simulink model "Model_1"  (R2020b)
settings: Solver=VariableStepAuto  StartTime=0.0  StopTime=200  RelTol=1e-3
settings Model: Creator=samar  LastModifiedBy=samar

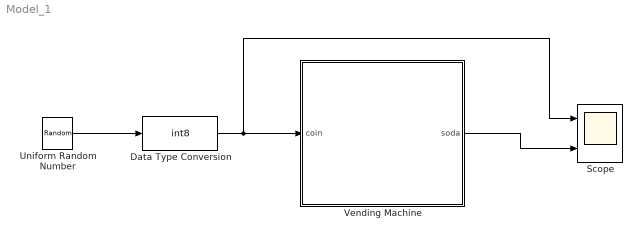
== system Model_1 ==
  Data Type Conversion : DataTypeConversion  OutDataTypeStr=int8  RndMeth=Nearest
  Scope : Scope  NumInputPorts=2
  Uniform Random Number : UniformRandomNumber  Minimum=0  Maximum=2  Seed=337  SampleTime=10
  Vending Machine : Stateflow chart  TreatAsAtomicUnit=on
  wires:
  Uniform Random Number/1 -> Data Type Conversion/1
  Data Type Conversion/1 -> Scope/1, Vending Machine/1(coin)
  Vending Machine/1(soda) -> Scope/2

== stateflow chart Model_1/Vending Machine ==
  state Default
  state Nickel_Coin
  state Dime_Coin
  (default) -> Default
  Default -> Nickel_Coin [order 1] : [coin==1]{soda=0}
  Nickel_Coin -> Default [order 2] : [coin==2]{soda=1}
  Dime_Coin -> Default [order 1] : [coin==1]{soda=1}
  Default -> Dime_Coin [order 2] : [coin==2]{soda=0}
  Nickel_Coin -> Dime_Coin [order 1] : [coin==1]{soda=0}
  Dime_Coin -> Nickel_Coin [order 2] : [coin==2]{soda=1}
  data: coin input; soda output
